simulink model "test"  (R2019a)
settings: Solver=VariableStepAuto  StartTime=0.0  StopTime=100  RelTol=1e-3
settings Model: Creator=ali  LastModifiedBy=ali

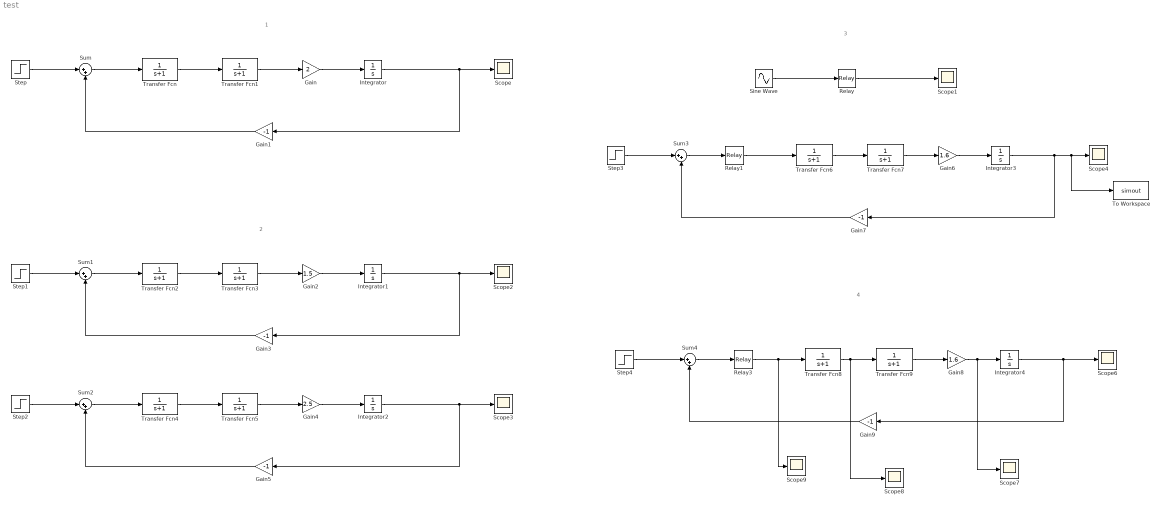
== system test ==
  note: 1
  note: 2
  note: 3
  note: 4
  Gain : Gain  Gain=2
  Gain{1,3,5,7,9} (5 alike) : Gain  Gain=-1
  Gain2 : Gain  Gain=1.5
  Gain4 : Gain  Gain=2.5
  Gain6 : Gain  Gain=1.6
  Gain8 : Gain  Gain=1.6
  Integrator{,1..4} (5 alike) : Integrator
  Relay : Relay  OnSwitchValue=0  OffSwitchValue=0  OnOutputValue=5  OffOutputValue=-5
  Relay1 : Relay  OnSwitchValue=0  OffSwitchValue=0  OnOutputValue=5  OffOutputValue=-5
  Relay3 : Relay  OnSwitchValue=5  OffSwitchValue=-5  OnOutputValue=5  OffOutputValue=-5
  Scope{,1..4,6..9} (9 alike) : Scope
  Sine Wave : Sin  SampleTime=0
  Step{,1..4} (5 alike) : Step  Before=1  After=0  SampleTime=0
  Sum{,1..4} (5 alike) : Sum  Inputs=|++
  To Workspace : ToWorkspace  VariableName=simout  SaveFormat=Timeseries  SampleTime=-1
  Transfer Fcn{,1..9} (10 alike) : TransferFcn  Denominator=[1 1]
  wires:
  Integrator/1 -> Scope/1, Gain1/1
  Sum/1 -> Transfer Fcn/1
  Gain1/1 -> Sum/2
  Transfer Fcn/1 -> Transfer Fcn1/1
  Transfer Fcn1/1 -> Gain/1
  Gain/1 -> Integrator/1
  Step/1 -> Sum/1
  Sine Wave/1 -> Relay/1
  Relay/1 -> Scope1/1
  Transfer Fcn2/1 -> Transfer Fcn3/1
  Sum1/1 -> Transfer Fcn2/1
  Gain3/1 -> Sum1/2
  Step1/1 -> Sum1/1
  Transfer Fcn3/1 -> Gain2/1
  Gain2/1 -> Integrator1/1
  Integrator1/1 -> Scope2/1, Gain3/1
  Transfer Fcn4/1 -> Transfer Fcn5/1
  Sum2/1 -> Transfer Fcn4/1
  Gain5/1 -> Sum2/2
  Step2/1 -> Sum2/1
  Transfer Fcn5/1 -> Gain4/1
  Gain4/1 -> Integrator2/1
  Integrator2/1 -> Scope3/1, Gain5/1
  Transfer Fcn6/1 -> Transfer Fcn7/1
  Gain7/1 -> Sum3/2
  Step3/1 -> Sum3/1
  Transfer Fcn7/1 -> Gain6/1
  Gain6/1 -> Integrator3/1
  Integrator3/1 -> To Workspace/1, Scope4/1, Gain7/1
  Sum3/1 -> Relay1/1
  Relay1/1 -> Transfer Fcn6/1
  Gain9/1 -> Sum4/2
  Step4/1 -> Sum4/1
  Gain8/1 -> Scope7/1, Integrator4/1
  Transfer Fcn9/1 -> Gain8/1
  Transfer Fcn8/1 -> Scope8/1, Transfer Fcn9/1
  Integrator4/1 -> Scope6/1, Gain9/1
  Relay3/1 -> Scope9/1, Transfer Fcn8/1
  Sum4/1 -> Relay3/1
